simulink model "q4d"  (R2024a)
settings: Solver=FixedStepAuto  StartTime=0.0  StopTime=65  FixedStep=1  RelTol=1e-3  EnableMultiTasking=on
settings Model: ExtModeTrigDuration=2  Creator=amir  LastModifiedBy=amir
settings SolverCC: AutoInsertRateTranBlk=on
settings OptimizationCC: DefaultParameterBehavior=Inlined  UseDivisionForNetSlopeComputation=on  GainParamInheritBuiltInType=on  UseFloatMulNetSlope=on  InlineInvariantSignals=on  PassReuseOutputArgsAs=Individual arguments  ZeroExternalMemoryAtStartup=off  ZeroInternalMemoryAtStartup=off  NoFixptDivByZeroProtection=on  EfficientFloat2IntCast=on  LifeSpan=1  MaxStackSize=64  OptimizeBlockOrder=speed  DifferentSizesBufferReuse=on  EfficientTunableParamExpr=on
settings DebuggingCC: ParameterTunabilityLossMsg=error
settings HardwareCC: ProdBitPerInt=16  ProdBitPerPointer=16  ProdBitPerSizeT=16  ProdBitPerPtrDiffT=16  ProdLargestAtomicFloat=None  ProdWordSize=8  ProdLongLongMode=on  ProdHWDeviceType=Atmel->AVR
settings SFSimCC: MATLABDynamicMemAlloc=off
settings RTWCC: Description=Embedded Coder  SystemTargetFile=ert.tlc  HardwareBoard=Arduino Uno  GenCodeOnly=on  TemplateMakefile=ert_default_tmf  GenerateReport=on  Toolchain=Arduino AVR  BuildConfiguration=Faster Runs  LaunchReport=on
settings CodeAppCC: ForceParamTrailComments=on  IgnoreCustomStorageClasses=off  OperatorAnnotations=on  SimulinkDataObjDesc=on  SFDataObjDesc=on  CustomSymbolStrGlobalVar=rt$N$M  CustomSymbolStrType=$N$M  CustomSymbolStrFcn=$N$M$F  CustomSymbolStrMacro=$N$M  InsertBlockDesc=on
settings ERTTargetCC: IncludeMdlTerminateFcn=off  CombineSignalStateStructs=on  SupportComplex=off  SupportNonInlinedSFcns=on  ExtModeTransport=3  ExtModeStaticAlloc=on  ExtModeAutomaticAllocSize=off  ExtModeStaticAllocSize=250  ExtModeMexFile=ext_xcp  ExtModeIntrfLevel=Level2 - Open  InlinedParameterPlacement=NonHierarchical  ERTFilePackagingFormat=CompactWithDataFile

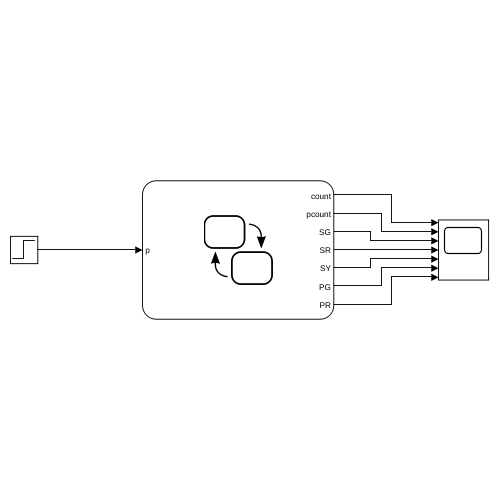
[thumbnail: Simulink's stored preview of the top-level diagram]
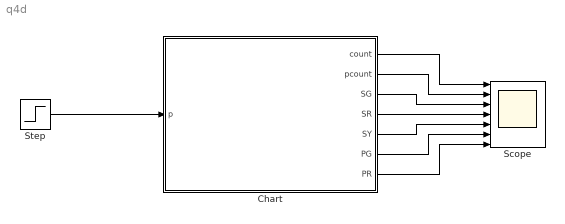
== system q4d ==
  Chart : Stateflow chart  TreatAsAtomicUnit=on
  Scope : Scope  NumInputPorts=7
  Step : Step  SampleTime=0
  wires:
  Chart/1(count) -> Scope/1
  Chart/2(pcount) -> Scope/2
  Step/1 -> Chart/1(p)
  Chart/3(SG) -> Scope/3
  Chart/4(SR) -> Scope/4
  Chart/5(SY) -> Scope/5
  Chart/6(PG) -> Scope/6
  Chart/7(PR) -> Scope/7

== stateflow chart q4d/Chart ==
  state carred_pedred
  state cargreen_pedred
  state carred_pedgreen
  state caryellow_pedred
  state pending_pedred
  cargreen_pedred -> cargreen_pedred [order 1] : [count<60]{count=count+1;}
  carred_pedred -> carred_pedred [order 2] : /{count=count+1;}
  (default) -> carred_pedgreen : {count=0; pcount=0; SR=1; PG=1;}
  carred_pedgreen -> carred_pedgreen [order 2] : {count=count+1; pcount=pcount+1;}
  cargreen_pedred -> caryellow_pedred [order 3] : [p && count>=60]{count=0; SY=1; SG=0;}
  carred_pedgreen -> carred_pedred [order 1] : [pcount>=55]{count=count+1; PR=1; PG=0;}
  carred_pedred -> cargreen_pedred [order 1] : [count>=60]{count=count+1; SG=1; SR=0;}
  cargreen_pedred -> pending_pedred [order 2] : [p==1 && count<60]
  caryellow_pedred -> carred_pedgreen [order 1] : [pcount>=5]{count=0; pcount=0; SR=1; PG=1; SY=0; PR=0;}
  pending_pedred -> caryellow_pedred [order 1] : [count>=60]{count=0; SY=1; SG=0;}
  caryellow_pedred -> caryellow_pedred [order 2] : {count=count+1;}
  pending_pedred -> pending_pedred [order 2] : {count=count+1}
  data: p input; count output; pcount output; SG output; SR output; SY output; PG output; PR output
